simulink model "gm_FCS_MPC_switching_states_6Phase_2level_inverter"  (R2022a)
settings: Solver=FixedStepDiscrete  StartTime=0.0  StopTime=10.0  RelTol=1e-3
undefined symbols (not defined in the file or in its folder): f_c
libraries: hdlmdlgenlib x12
settings Model: Creator=Andre Merx  LastModifiedBy=Andre Merx
settings SolverCC: AlgebraicLoopSolver=TrustRegion
settings DataIOCC: LimitDataPoints=on  SaveOutput=off  SaveTime=off
settings OptimizationCC: BlockReduction=off  ConditionallyExecuteInputs=off  DefaultParameterBehavior=Inlined  LifeSpan=inf
settings DebuggingCC: AlgebraicLoopMsg=error  InheritedTsInSrcMsg=none  SingleTaskRateTransMsg=error  UnconnectedInputMsg=warning  UnconnectedOutputMsg=warning  UnconnectedLineMsg=warning  AllowSymbolicDim=off  StrictBusMsg=ErrorOnBusTreatedAsVector  SFUnexpectedBacktrackingDiag=warning  SFNoUnconditionalDefaultTransitionDiag=warning  SFExecutionAtInitializationDiag=none  SFMachineParentedDataDiag=warning  ArithmeticOperatorsInVariantConditions=warning
settings HardwareCC: ProdBitPerPointer=32  ProdBitPerSizeT=32  ProdBitPerPtrDiffT=32  ProdLargestAtomicFloat=None  ProdIntDivRoundTo=Undefined  ProdEndianess=Unspecified  ProdWordSize=32  ProdHWDeviceType=ASIC/FPGA->ASIC/FPGA  ProdEqTarget=off
settings SFSimCC: SimUseLocalCustomCode=off  CustomCodeUndefinedFunction=UseInterfaceOnly
settings RTWCC: RTWUseLocalCustomCode=off
settings CodeAppCC: StateflowObjectComments=on
settings GRTTargetCC: TargetLangStandard=C89/C90 (ANSI)
settings ConfigComp: CovScope=ReferencedModels  CovMetricSettings=dw  CovSaveCumulativeToWorkspaceVar=on  CovSaveSingleToWorkspaceVar=on  CovExternalEMLEnable=off  CovSFcnEnable=off

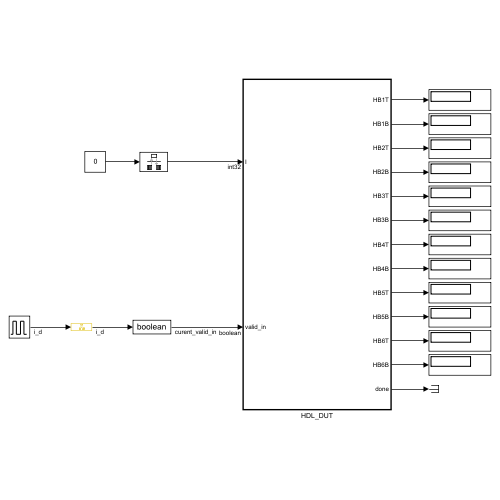
[thumbnail: Simulink's stored preview of the top-level diagram]
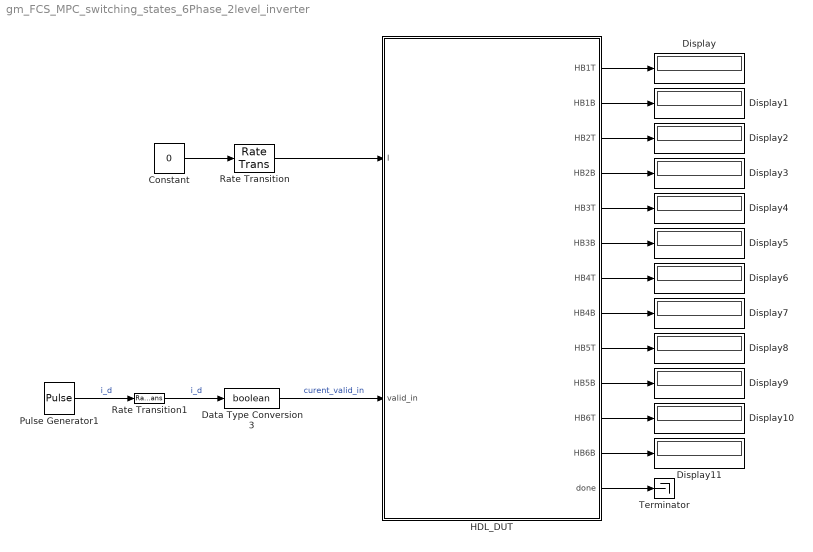
== system gm_FCS_MPC_switching_states_6Phase_2level_inverter ==
  Constant : Constant  Value=0  OutDataTypeStr=int32  SampleTime=-1
  Data Type Conversion3 : DataTypeConversion  OutDataTypeStr=boolean  SaturateOnIntegerOverflow=off  RndMeth=Floor
  Display{,1..11} (12 alike) : Display
  HDL_DUT : Subsystem  TreatAsAtomicUnit=on
  Pulse Generator1 : DiscretePulseGenerator  PulseType=Time based  Period=1/f_c
  Rate Transition : RateTransition  OutPortSampleTime=Rt
  Rate Transition1 : RateTransition  OutPortSampleTime=Rt
  Terminator : Terminator
  wires:
  HDL_DUT/13(done) -> Terminator/1
  HDL_DUT/12(HB6B) -> Display11/1
  HDL_DUT/11(HB6T) -> Display10/1
  HDL_DUT/10(HB5B) -> Display9/1
  HDL_DUT/9(HB5T) -> Display8/1
  HDL_DUT/8(HB4B) -> Display7/1
  HDL_DUT/7(HB4T) -> Display6/1
  HDL_DUT/6(HB3B) -> Display5/1
  HDL_DUT/5(HB3T) -> Display4/1
  HDL_DUT/4(HB2B) -> Display3/1
  HDL_DUT/3(HB2T) -> Display2/1
  HDL_DUT/2(HB1B) -> Display1/1
  HDL_DUT/1(HB1T) -> Display/1
  Data Type Conversion3/1 -> HDL_DUT/2(valid_in)  "curent_valid_in"
  Pulse Generator1/1 -> Rate Transition1/1  "i_d"
  Rate Transition1/1 -> Data Type Conversion3/1  "i_d"
  Rate Transition/1 -> HDL_DUT/1(I)
  Constant/1 -> Rate Transition/1

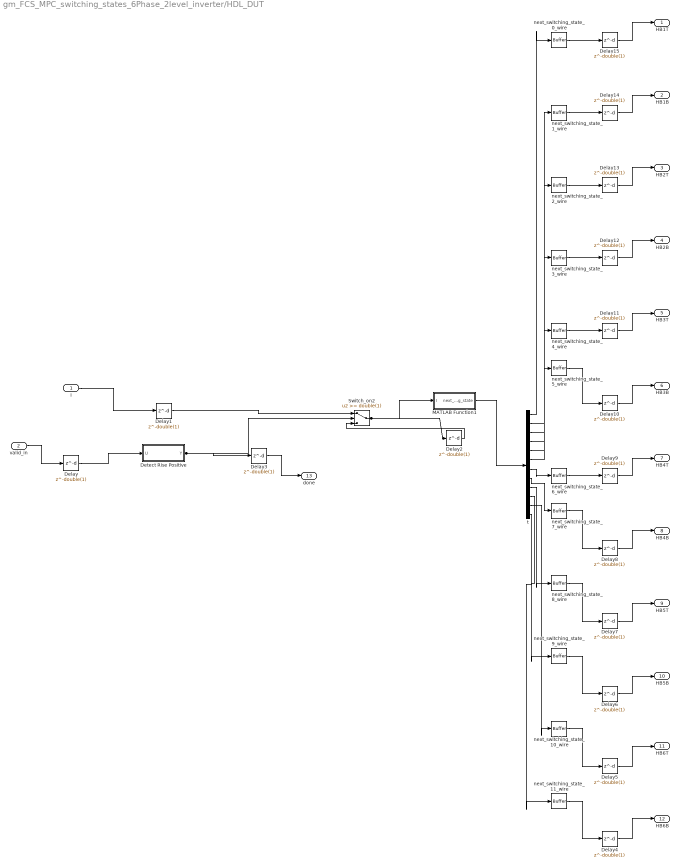
== system gm_FCS_MPC_switching_states_6Phase_2level_inverter/HDL_DUT ==
  I : Inport  OutDataTypeStr=int32  PortDimensions=1  SampleTime=1e-08
  valid_in : Inport  Port=2  OutDataTypeStr=boolean  PortDimensions=1  SampleTime=1e-08
  Delay{,1..15} (16 alike) : Delay  DelayLength=double(1)  InitialCondition=0  SampleTime=1e-08
  Detect Rise Positive : Subsystem  mask(Detect Rise Positive){vinit=double(0), InputProcessing=Elements as channels (sample based), OutDataTypeStr=boolean}
      mask prompts: vinit "Simulink:masks:InitialCondition_MP"; InputProcessing "Simulink:masks:InputProcessing_MP"; OutDataTypeStr "Simulink:masks:OutputDataType_MP"
      mask help: Simulink:masks:DetectRisePositive_MD
      mask init:
      | InputProcessing = 'Elements as channels (sample based)';
      | OutDataTypeStr = 'boolean';
      | vinit = double(0);
      mask TypeOptions InputProcessing: Simulink:masks:ColumnsAsChannelsFrameBased | Simulink:masks:ElementsAsChannelsSampleBased
      mask TypeOptions OutDataTypeStr: Simulink:masks:uint8 | Simulink:masks:boolean
      mask Display: fprintf('U > 0\n&  NOT\nU/z > 0')
  MATLAB Function1 : Subsystem
  Switch_on2 : Switch  Threshold=double(1)  OutDataTypeStr=int32  RndMeth=Simplest  SampleTime=1e-08  SaturateOnIntegerOverflow=off  InputSameDT=off
  next_switching_state_0_wire : hdlmdlgenlib/Buffer
      settings: SourceProductBaseCode=SL
  next_switching_state_10_wire : hdlmdlgenlib/Buffer
      settings: SourceProductBaseCode=SL
  next_switching_state_11_wire : hdlmdlgenlib/Buffer
      settings: SourceProductBaseCode=SL
  next_switching_state_1_wire : hdlmdlgenlib/Buffer
      settings: SourceProductBaseCode=SL
  next_switching_state_2_wire : hdlmdlgenlib/Buffer
      settings: SourceProductBaseCode=SL
  next_switching_state_3_wire : hdlmdlgenlib/Buffer
      settings: SourceProductBaseCode=SL
  next_switching_state_4_wire : hdlmdlgenlib/Buffer
      settings: SourceProductBaseCode=SL
  next_switching_state_5_wire : hdlmdlgenlib/Buffer
      settings: SourceProductBaseCode=SL
  next_switching_state_6_wire : hdlmdlgenlib/Buffer
      settings: SourceProductBaseCode=SL
  next_switching_state_7_wire : hdlmdlgenlib/Buffer
      settings: SourceProductBaseCode=SL
  next_switching_state_8_wire : hdlmdlgenlib/Buffer
      settings: SourceProductBaseCode=SL
  next_switching_state_9_wire : hdlmdlgenlib/Buffer
      settings: SourceProductBaseCode=SL
  t : Demux  Outputs=12
  HB1T : Outport  SampleTime=1e-08
  HB1B : Outport  Port=2  SampleTime=1e-08
  HB2T : Outport  Port=3  SampleTime=1e-08
  HB2B : Outport  Port=4  SampleTime=1e-08
  HB3T : Outport  Port=5  SampleTime=1e-08
  HB3B : Outport  Port=6  SampleTime=1e-08
  HB4T : Outport  Port=7  SampleTime=1e-08
  HB4B : Outport  Port=8  SampleTime=1e-08
  HB5T : Outport  Port=9  SampleTime=1e-08
  HB5B : Outport  Port=10  SampleTime=1e-08
  HB6T : Outport  Port=11  SampleTime=1e-08
  HB6B : Outport  Port=12  SampleTime=1e-08
  done : Outport  Port=13  SampleTime=1e-08
  wires:
  I/1 -> Delay1/1
  valid_in/1 -> Delay/1
  Delay/1 -> Detect Rise Positive/1(U)
  Delay1/1 -> Switch_on2/1
  Delay10/1 -> HB3B/1
  Delay11/1 -> HB3T/1
  Delay12/1 -> HB2B/1
  Delay13/1 -> HB2T/1
  Delay14/1 -> HB1B/1
  Delay15/1 -> HB1T/1
  Delay2/1 -> Switch_on2/3
  Delay3/1 -> done/1
  Delay4/1 -> HB6B/1
  Delay5/1 -> HB6T/1
  Delay6/1 -> HB5B/1
  Delay7/1 -> HB5T/1
  Delay8/1 -> HB4B/1
  Delay9/1 -> HB4T/1
  next_switching_state_0_wire/1 -> Delay15/1
  next_switching_state_1_wire/1 -> Delay14/1
  next_switching_state_2_wire/1 -> Delay13/1
  next_switching_state_3_wire/1 -> Delay12/1
  next_switching_state_4_wire/1 -> Delay11/1
  next_switching_state_5_wire/1 -> Delay10/1
  next_switching_state_6_wire/1 -> Delay9/1
  next_switching_state_7_wire/1 -> Delay8/1
  next_switching_state_8_wire/1 -> Delay7/1
  next_switching_state_9_wire/1 -> Delay6/1
  next_switching_state_10_wire/1 -> Delay5/1
  next_switching_state_11_wire/1 -> Delay4/1
  Detect Rise Positive/1(Y) -> Switch_on2/2, Delay3/1
  MATLAB Function1/1(next_switching_state) -> t/1
  Switch_on2/1 -> Delay2/1, MATLAB Function1/1(I)
  t/1 -> next_switching_state_0_wire/1
  t/2 -> next_switching_state_1_wire/1
  t/3 -> next_switching_state_2_wire/1
  t/4 -> next_switching_state_3_wire/1
  t/5 -> next_switching_state_4_wire/1
  t/6 -> next_switching_state_5_wire/1
  t/7 -> next_switching_state_6_wire/1
  t/8 -> next_switching_state_7_wire/1
  t/9 -> next_switching_state_8_wire/1
  t/10 -> next_switching_state_9_wire/1
  t/11 -> next_switching_state_10_wire/1
  t/12 -> next_switching_state_11_wire/1

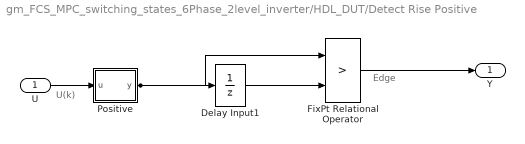
== system gm_FCS_MPC_switching_states_6Phase_2level_inverter/HDL_DUT/Detect Rise Positive ==
  note: Edge
  note: U(k)
  U : Inport  OutDataTypeStr=boolean  SampleTime=1e-08
  Delay Input1 : UnitDelay  Description=Store in Global RAM  DisableCoverage=on  InitialCondition=vinit  SampleTime=-1  HasFrameUpgradeWarning=on
  FixPt Relational Operator : RelationalOperator  Operator=>  OutDataTypeStr=boolean  ZeroCross=off  InputSameDT=off
  Positive : Subsystem  mask(Compare To Zero){relop=>, OutDataTypeStr=boolean, ZeroCross=off}
      mask prompts: relop "Simulink:masks:Operator_MP"; OutDataTypeStr "Simulink:masks:OutputDataType_MP"; ZeroCross "Simulink:masks:EnableZerocrossingDetection_MP"
      mask help: Simulink:masks:CompareToZero_MD
      mask init:
      | OutDataTypeStr = 'boolean';
      | ZeroCross = 'off';
      | blkName = 'FCS_MPC_switching_states_6Phase_2level_inverter/HDL_DUT/Detect Rise\nPositive/Positive';
      | relop = '>';
      | setValue = 'boolean';
      mask TypeOptions relop: == | ~= | < | <= | >= | >
      mask TypeOptions OutDataTypeStr: Simulink:masks:uint8 | Simulink:masks:boolean
      mask Callback ZeroCross: sl('zeroCrossEnable', gcbh);
      mask Display: disp([relop,' 0'])
  Y : Outport  SampleTime=1e-08
  wires:
  U/1 -> Positive/1(u)
  Delay Input1/1 -> FixPt Relational Operator/2
  FixPt Relational Operator/1 -> Y/1
  Positive/1(y) -> FixPt Relational Operator/1, Delay Input1/1

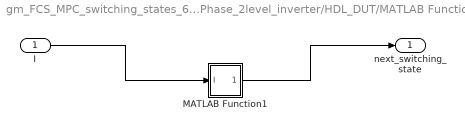
== system gm_FCS_MPC_switching_states_6Phase_2level_inverter/HDL_DUT/MATLAB Function1 ==
  I : Inport  OutDataTypeStr=int32  PortDimensions=1  SampleTime=1e-08
  MATLAB Function1 : MATLAB Function  TreatAsAtomicUnit=on
  next_switching_state : Outport  SampleTime=1e-08  VectorParamsAs1DForOutWhenUnconnected=off
  wires:
  I/1 -> MATLAB Function1/1(I)
  MATLAB Function1/1(next_switching_state) -> next_switching_state/1

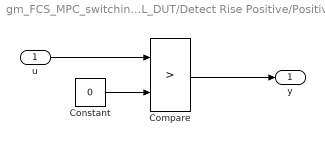
== system gm_FCS_MPC_switching_states_6Phase_2level_inverter/HDL_DUT/Detect Rise Positive/Positive ==
  u : Inport  OutDataTypeStr=boolean  SampleTime=1e-08
  Compare : RelationalOperator  Operator=>  OutDataTypeStr=boolean  ZeroCross=off
  Constant : Constant  DisableCoverage=on  Value=0  OutDataTypeStr=Inherit: Inherit via back propagation  SampleTime=-1  PreserveConstantTs=on
  y : Outport  SampleTime=1e-08
  wires:
  u/1 -> Compare/1
  Compare/1 -> y/1
  Constant/1 -> Compare/2

== matlab function gm_FCS_MPC_switching_states_6Phase_2level_inverter/HDL_DUT/MATLAB Function1/MATLAB Function1 ==
  data: I input; next_switching_state output
function next_switching_state = fcn(I)

    % Possible switching states of the 6-Phase 2-level inverter
    possible_swichting_states = [0	1	0	1	0	1	0	1	0	1	0	1;
                                1	0	0	1	0	1	0	1	0	1	0	1;
                                0	1	1	0	0	1	0	1	0	1	0	1;
                                1	0	1	0	0	1	0	1	0	1	0	1;
                                0	1	0	1	1	0	0	1	0	1	0	1;
                                1	0	0	1	1	0	0	1	0	1	0	1;
                                0	1	1	0	1	0	0	1	0	1	0	1;
                                1	0	1	0	1	0	0	1	0	1	0	1;
                                0	1	0	1	0	1	1	0	0	1	0	1;
                                1	0	0	1	0	1	1	0	0	1	0	1;
                                0	1	1	0	0	1	1	0	0	1	0	1;
                                1	0	1	0	0	1	1	0	0	1	0	1;
                                0	1	0	1	1	0	1	0	0	1	0	1;
                                1	0	0	1	1	0	1	0	0	1	0	1;
                                0	1	1	0	1	0	1	0	0	1	0	1;
                                1	0	1	0	1	0	1	0	0	1	0	1;
                                0	1	0	1	0	1	0	1	1	0	0	1;
                                1	0	0	1	0	1	0	1	1	0	0	1;
                                0	1	1	0	0	1	0	1	1	0	0	1;
                                1	0	1	0	0	1	0	1	1	0	0	1;
                                0	1	0	1	1	0	0	1	1	0	0	1;
                                1	0	0	1	1	0	0	1	1	0	0	1;
                                0	1	1	0	1	0	0	1	1	0	0	1;
                                1	0	1	0	1	0	0	1	1	0	0	1;
                                0	1	0	1	0	1	1	0	1	0	0	1;
                                1	0	0	1	0	1	1	0	1	0	0	1;
                                0	1	1	0	0	1	1	0	1	0	0	1;
                                1	0	1	0	0	1	1	0	1	0	0	1;
                                0	1	0	1	1	0	1	0	1	0	0	1;
                                1	0	0	1	1	0	1	0	1	0	0	1;
                                0	1	1	0	1	0	1	0	1	0	0	1;
                                1	0	1	0	1	0	1	0	1	0	0	1;
                                0	1	0	1	0	1	0	1	0	1	1	0;
                                1	0	0	1	0	1	0	1	0	1	1	0;
                                0	1	1	0	0	1	0	1	0	1	1	0;
                                1	0	1	0	0	1	0	1	0	1	1	0;
                                0	1	0	1	1	0	0	1	0	1	1	0;
                                1	0	0	1	1	0	0	1	0	1	1	0;
                                0	1	1	0	1	0	0	1	0	1	1	0;
                                1	0	1	0	1	0	0	1	0	1	1	0;
                                0	1	0	1	0	1	1	0	0	1	1	0;
                                1	0	0	1	0	1	1	0	0	1	1	0;
                                0	1	1	0	0	1	1	0	0	1	1	0;
                                1	0	1	0	0	1	1	0	0	1	1	0;
                                0	1	0	1	1	0	1	0	0	1	1	0;
                                1	0	0	1	1	0	1	0	0	1	1	0;
                                0	1	1	0	1	0	1	0	0	1	1	0;
                                1	0	1	0	1	0	1	0	0	1	1	0;
                                0	1	0	1	0	1	0	1	1	0	1	0;
                                1	0	0	1	0	1	0	1	1	0	1	0;
                                0	1	1	0	0	1	0	1	1	0	1	0;
                                1	0	1	0	0	1	0	1	1	0	1	0;
                                0	1	0	1	1	0	0	1	1	0	1	0;
                                1	0	0	1	1	0	0	1	1	0	1	0;
                                0	1	1	0	1	0	0	1	1	0	1	0;
                                1	0	1	0	1	0	0	1	1	0	1	0;
                                0	1	0	1	0	1	1	0	1	0	1	0;
                                1	0	0	1	0	1	1	0	1	0	1	0;
                                0	1	1	0	0	1	1	0	1	0	1	0;
                                1	0	1	0	0	1	1	0	1	0	1	0;
                                0	1	0	1	1	0	1	0	1	0	1	0;
                                1	0	0	1	1	0	1	0	1	0	1	0;
                                0	1	1	0	1	0	1	0	1	0	1	0;
                                1	0	1	0	1	0	1	0	1	0	1	0];

    % Initial condition
    if I==0
        I=int32(1);
    end

    % Output switching state
    next_switching_state=boolean(possible_swichting_states(I,:))';

end
